simulink model "M_MSGPACKER"  (R2022a)
settings: Solver=ode4  StartTime=0.0  StopTime=0.04  FixedStep=0.04  RelTol=1e-3
PreLoadFcn:
  | listing = dir;
  | if (contains([listing .name], 'M_MSGPACKER.slx'))
  |     addpath('./DYN', './FLCC', './FTG', './GPS', './INS', './MAP', './RALT');
  | elseif (contains([listing .name], 'FTG.slx'))
  |     addpath('../DYN', '../FLCC', '../FTG', '../GPS', '../INS', '../MAP', '../RALT');
  | else
  | 
  | end
  | 
  | load('BUS_STRUCTURE_RALT.mat');
  | load('BUS_STRUCTURE_INS.mat');
  | load('BUS_STRUCTURE_GPS.mat');
InitFcn:
  | listing = dir;
  | if (contains([listing .name], 'M_MSGPACKER'))
  |     addpath('./DYN', './FLCC', './FTG', './GPS', './INS', './MAP', './RALT');
  | elseif (contains([listing .name], 'FTG.slx'))
  |     addpath('../DYN', '../FLCC', '../FTG', '../GPS', '../INS', '../MAP', '../RALT');
  | else
  | 
  | end
  | 
  | load('BUS_STRUCTURE_RALT.mat');
  | load('BUS_STRUCTURE_INS.mat');
  | load('BUS_STRUCTURE_GPS.mat');
undefined symbols (not defined in the file or in its folder): ft, m, s
libraries: aerolibconvert2 x14, simulink_extras x5
settings Model: Creator=ASCL  LastModifiedBy=ASCL
settings DataIOCC: SaveOutput=off  DSMLogging=off  SaveTime=off
settings OptimizationCC: BlockReduction=off  DefaultParameterBehavior=Inlined  UseDivisionForNetSlopeComputation=on  GainParamInheritBuiltInType=on  UseFloatMulNetSlope=on  ExpressionFolding=off  PassReuseOutputArgsAs=Individual arguments  ZeroExternalMemoryAtStartup=off  ZeroInternalMemoryAtStartup=off  EfficientFloat2IntCast=on  LifeSpan=inf  OptimizeBlockOrder=speed  DifferentSizesBufferReuse=on  EfficientTunableParamExpr=on
settings DebuggingCC: SignalInfNanChecking=warning  ReadBeforeWriteMsg=EnableAllAsError  WriteAfterWriteMsg=EnableAllAsError  WriteAfterReadMsg=EnableAllAsError  IntegerOverflowMsg=error  ParameterTunabilityLossMsg=error  UniqueDataStoreMsg=error  AssertControl=DisableAll  NonBusSignalsTreatedAsBus=error  SFInvalidInputDataAccessInChartInitDiag=error  SFTransitionOutsideNaturalParentDiag=error  SFUnreachableExecutionPathDiag=error  SFUndirectedBroadcastEventsDiag=error  IntegerSaturationMsg=error
settings HardwareCC: ProdBitPerPointer=32  ProdBitPerSizeT=32  ProdBitPerPtrDiffT=32  ProdLargestAtomicInteger=Long  ProdLargestAtomicFloat=Double  ProdEndianess=BigEndian  ProdWordSize=32  ProdLongLongMode=on  ProdHWDeviceType=Freescale->MPC83xx
settings ModelReferenceCC: ModelReferenceNumInstancesAllowed=Single
settings SFSimCC: CompileTimeRecursionLimit=0  EnableRuntimeRecursion=off  MATLABDynamicMemAlloc=off
settings RTWCC: SystemTargetFile=ert.tlc  TemplateMakefile=ert_default_tmf  GenerateReport=on  RTWUseSimCustomCode=on  BuildConfiguration=Faster Runs  IncludeHyperlinkInReport=on  LaunchReport=on  GenerateTraceInfo=on  GenerateTraceReport=on  GenerateTraceReportSl=on  GenerateTraceReportSf=on  GenerateTraceReportEml=on  GenerateCodeMetricsReport=on
settings CodeAppCC: ForceParamTrailComments=on  IgnoreCustomStorageClasses=off  OperatorAnnotations=on  SimulinkDataObjDesc=on  SFDataObjDesc=on  MATLABFcnDesc=on  InsertBlockDesc=on  StateflowObjectComments=on  MATLABSourceComments=on  EnableCustomComments=on  InlinedPrmAccess=Macros  ReqsInCode=on
settings ERTTargetCC: TargetLangStandard=C99 (ISO)  UtilityFuncGeneration=Shared location  GenerateSampleERTMain=on  IncludeMdlTerminateFcn=off  CombineSignalStateStructs=on  SuppressErrorStatus=on  SupportAbsoluteTime=off  SupportNonFinite=off  SupportComplex=off  ParenthesesLevel=Standards  CastingMode=Standards  GenerateSharedConstants=off  InlinedParameterPlacement=NonHierarchical  ERTCustomFileTemplate=example_file_process.tlc  RateTransitionBlockCode=Function  PreserveIfCondition=on  ConvertIfToSwitch=off  EnableSignedLeftShifts=off  EnableSignedRightShifts=off

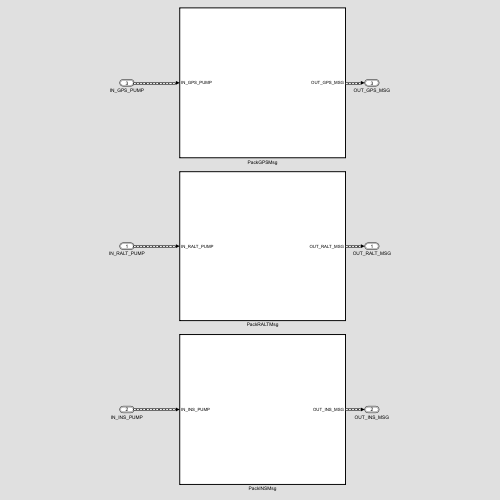
[thumbnail: Simulink's stored preview of the top-level diagram]
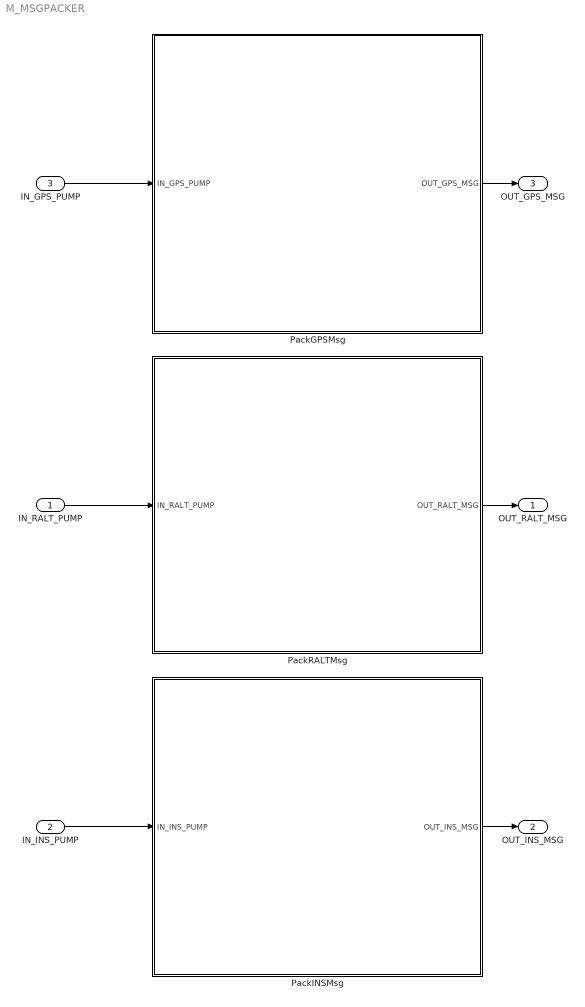
== system M_MSGPACKER ==
  IN_RALT_PUMP : Inport  OutDataTypeStr=Bus: BUS_SENSOR_RALT_DP  SampleTime=0.04  Interpolate=off  BusOutputAsStruct=on
  IN_INS_PUMP : Inport  Port=2  OutDataTypeStr=Bus: BUS_SENSOR_INS_DP  SampleTime=0.04  Interpolate=off  BusOutputAsStruct=on
  IN_GPS_PUMP : Inport  Port=3  OutDataTypeStr=Bus: BUS_SENSOR_GPS_DP  SampleTime=0.04  Interpolate=off  BusOutputAsStruct=on
  PackGPSMsg : Subsystem  TreatAsAtomicUnit=on
      settings: RTWSystemCode=Nonreusable function  RTWFcnNameOpts=Use subsystem name  FunctionInterfaceSpec=Allow arguments (Match graphical interface)
  PackINSMsg : Subsystem  TreatAsAtomicUnit=on
      settings: RTWSystemCode=Nonreusable function  RTWFcnNameOpts=Use subsystem name  FunctionInterfaceSpec=Allow arguments (Match graphical interface)
  PackRALTMsg : Subsystem  TreatAsAtomicUnit=on
      settings: RTWSystemCode=Nonreusable function  RTWFcnNameOpts=Use subsystem name  FunctionInterfaceSpec=Allow arguments (Match graphical interface)
  OUT_RALT_MSG : Outport  OutDataTypeStr=Bus: BUS_SENSOR_RALT  SampleTime=0.04  BusOutputAsStruct=on
  OUT_INS_MSG : Outport  Port=2  OutDataTypeStr=Bus: BUS_SENSOR_INS  SampleTime=0.04  BusOutputAsStruct=on
  OUT_GPS_MSG : Outport  Port=3  OutDataTypeStr=Bus: BUS_SENSOR_GPS  SampleTime=0.04  BusOutputAsStruct=on
  wires:
  IN_INS_PUMP/1 -> PackINSMsg/1(IN_INS_PUMP)
  PackGPSMsg/1(OUT_GPS_MSG) -> OUT_GPS_MSG/1
  IN_GPS_PUMP/1 -> PackGPSMsg/1(IN_GPS_PUMP)
  PackINSMsg/1(OUT_INS_MSG) -> OUT_INS_MSG/1
  PackRALTMsg/1(OUT_RALT_MSG) -> OUT_RALT_MSG/1
  IN_RALT_PUMP/1 -> PackRALTMsg/1(IN_RALT_PUMP)

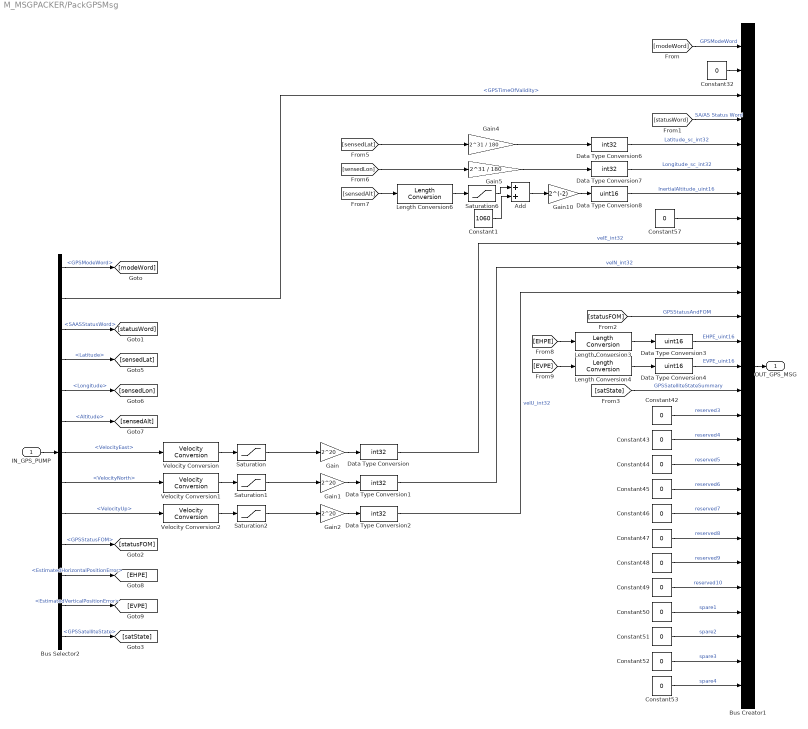
== system M_MSGPACKER/PackGPSMsg ==
  IN_GPS_PUMP : Inport  OutDataTypeStr=Bus: BUS_SENSOR_GPS_DP  SampleTime=0.04
  Add : Sum
  Bus Creator1 : BusCreator  Inputs=27  OutDataTypeStr=Bus: BUS_SENSOR_GPS  NonVirtualBus=on
      settings: InheritFromInputs=off
  Bus Selector2 : BusSelector  OutputSignals=GPSModeWord,GPSTimeOfValidity,SAASStatusWord,Latitude,Longitude,Altitude,VelocityEast,VelocityNorth,VelocityUp,GPSStatusFOM,EstimatedHorizontalPositionError,EstimatedVerticalPositionError,GPSSatelliteState
  Constant1 : Constant  Value=1060  SampleTime=0.04
  Constant{32,42..53,57} (14 alike) : Constant  Value=0  OutDataTypeStr=uint16  SampleTime=0.04
  Data Type Conversion{,1..2,6..7} (5 alike) : DataTypeConversion  OutDataTypeStr=int32  SaturateOnIntegerOverflow=off  RndMeth=Floor
  Data Type Conversion3 : DataTypeConversion  OutDataTypeStr=uint16  SaturateOnIntegerOverflow=off  RndMeth=Floor
  Data Type Conversion4 : DataTypeConversion  OutDataTypeStr=uint16  SaturateOnIntegerOverflow=off  RndMeth=Floor
  Data Type Conversion8 : DataTypeConversion  OutDataTypeStr=uint16  SaturateOnIntegerOverflow=off  RndMeth=Floor
  Gain : Gain  Gain=2^20
  Gain1 : Gain  Gain=2^20
  Gain10 : Gain  Gain=2^(-2)
  Gain2 : Gain  Gain=2^20
  Gain4 : Gain  Gain=2^31 / 180
  Gain5 : Gain  Gain=2^31 / 180
  Length Conversion3 : aerolibconvert2/Length Conversion  IU=m  OU=ft
  Length Conversion4 : aerolibconvert2/Length Conversion  IU=m  OU=ft
  Length Conversion6 : aerolibconvert2/Length Conversion  IU=m  OU=ft
  Saturation : Saturate  UpperLimit=2048  LowerLimit=-2048
  Saturation1 : Saturate  UpperLimit=2048  LowerLimit=-2048
  Saturation2 : Saturate  UpperLimit=2048  LowerLimit=-2048
  Saturation6 : Saturate  UpperLimit=80337  LowerLimit=-1060
  Velocity Conversion : aerolibconvert2/Velocity Conversion  IU=m/s  OU=ft/s
  Velocity Conversion1 : aerolibconvert2/Velocity Conversion  IU=m/s  OU=ft/s
  Velocity Conversion2 : aerolibconvert2/Velocity Conversion  IU=m/s  OU=ft/s
  OUT_GPS_MSG : Outport  SampleTime=0.04
  wires:
  Bus Creator1/1 -> OUT_GPS_MSG/1
  Data Type Conversion8/1 -> Bus Creator1/7  "InertialAltitude_uint16"
  Constant49/1 -> Bus Creator1/23  "reserved10"
  Gain4/1 -> Data Type Conversion6/1
  Constant44/1 -> Bus Creator1/18  "reserved5"
  [statusWord] -> Bus Creator1/4  "SA/AS Status Word"
  Gain5/1 -> Data Type Conversion7/1
  Constant1/1 -> Add/2
  Constant42/1 -> Bus Creator1/16  "reserved3"
  Constant46/1 -> Bus Creator1/20  "reserved7"
  Data Type Conversion4/1 -> Bus Creator1/14  "EVPE_uint16"
  Constant53/1 -> Bus Creator1/27  "spare4"
  Data Type Conversion3/1 -> Bus Creator1/13  "EHPE_uint16"
  Constant50/1 -> Bus Creator1/24  "spare1"
  [EVPE] -> Length Conversion4/1
  Velocity Conversion2/1 -> Saturation2/1
  Data Type Conversion6/1 -> Bus Creator1/5  "Latitude_sc_int32"
  Gain/1 -> Data Type Conversion/1
  [sensedLat] -> Gain4/1
  Constant52/1 -> Bus Creator1/26  "spare3"
  Constant47/1 -> Bus Creator1/21  "reserved8"
  Data Type Conversion7/1 -> Bus Creator1/6  "Longitude_sc_int32"
  Constant32/1 -> Bus Creator1/2
  Constant57/1 -> Bus Creator1/8
  Gain10/1 -> Data Type Conversion8/1
  Constant45/1 -> Bus Creator1/19  "reserved6"
  [satState] -> Bus Creator1/15  "GPSSatelliteStateSummary"
  Saturation6/1 -> Add/1
  Constant48/1 -> Bus Creator1/22  "reserved9"
  [statusFOM] -> Bus Creator1/12  "GPSStatusAndFOM"
  Gain1/1 -> Data Type Conversion1/1
  Velocity Conversion/1 -> Saturation/1
  Constant43/1 -> Bus Creator1/17  "reserved4"
  Length Conversion3/1 -> Data Type Conversion3/1
  Constant51/1 -> Bus Creator1/25  "spare2"
  Add/1 -> Gain10/1
  [sensedLon] -> Gain5/1
  Data Type Conversion/1 -> Bus Creator1/9  "velE_int32"
  Data Type Conversion2/1 -> Bus Creator1/11  "velU_int32"
  Data Type Conversion1/1 -> Bus Creator1/10  "velN_int32"
  Saturation1/1 -> Gain1/1
  Length Conversion4/1 -> Data Type Conversion4/1
  Gain2/1 -> Data Type Conversion2/1
  Velocity Conversion1/1 -> Saturation1/1
  Saturation2/1 -> Gain2/1
  [modeWord] -> Bus Creator1/1  "GPSModeWord"
  [sensedAlt] -> Length Conversion6/1
  Saturation/1 -> Gain/1
  [EHPE] -> Length Conversion3/1
  Length Conversion6/1 -> Saturation6/1
  IN_GPS_PUMP/1 -> Bus Selector2/1
  Bus Selector2/13 -> [satState]  "<GPSSatelliteState>"
  Bus Selector2/12 -> [EVPE]  "<EstimatedVerticalPositionError>"
  Bus Selector2/11 -> [EHPE]  "<EstimatedHorizontalPositionError>"
  Bus Selector2/10 -> [statusFOM]  "<GPSStatusFOM>"
  Bus Selector2/9 -> Velocity Conversion2/1  "<VelocityUp>"
  Bus Selector2/8 -> Velocity Conversion1/1  "<VelocityNorth>"
  Bus Selector2/7 -> Velocity Conversion/1  "<VelocityEast>"
  Bus Selector2/6 -> [sensedAlt]  "<Altitude>"
  Bus Selector2/5 -> [sensedLon]  "<Longitude>"
  Bus Selector2/4 -> [sensedLat]  "<Latitude>"
  Bus Selector2/3 -> [statusWord]  "<SAASStatusWord>"
  Bus Selector2/1 -> [modeWord]  "<GPSModeWord>"
  Bus Selector2/2 -> Bus Creator1/3  "<GPSTimeOfValidity>"

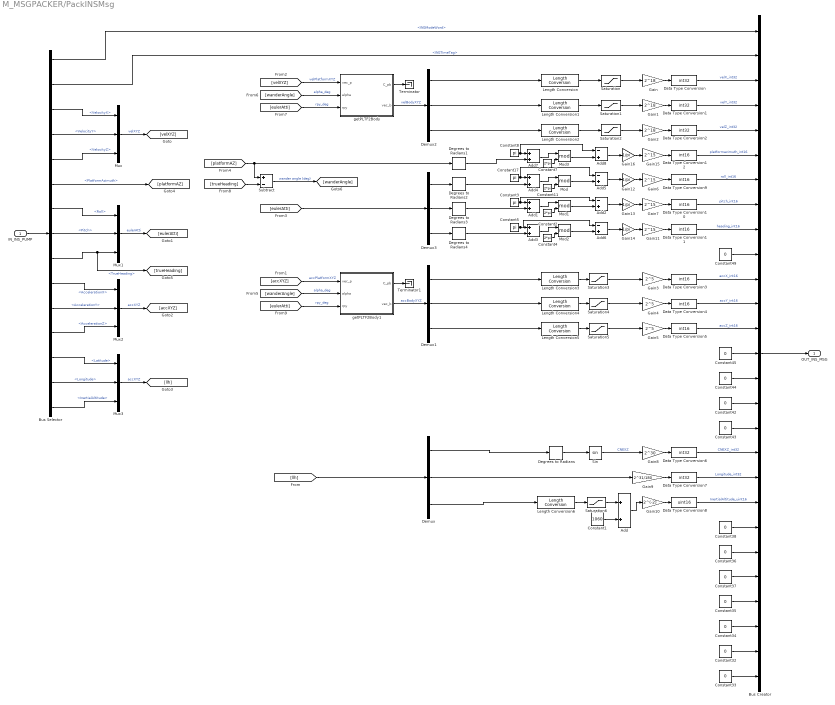
== system M_MSGPACKER/PackINSMsg ==
  IN_INS_PUMP : Inport  OutDataTypeStr=Bus: BUS_SENSOR_INS_DP  SampleTime=0.04
  Add{,1,3..4,7} (5 alike) : Sum
  Add{2,5..6,8} (4 alike) : Sum  Inputs=-+
  Bus Creator : BusCreator  Inputs=27  OutDataTypeStr=Bus: BUS_SENSOR_INS  NonVirtualBus=on
      settings: InheritFromInputs=off
  Bus Selector : BusSelector  OutputSignals=INSModeWord,INSTimeTag,VelocityX,VelocityY,VelocityZ,PlatformAzimuth,Roll,Pitch,TrueHeading,AccelerationX,AccelerationY,AccelerationZ,Latitude,Longitude,InertialAltitude
  Constant1 : Constant  Value=1060  SampleTime=0.04
  Constant{2,4,7,11} (4 alike) : Constant  Value=2*pi  SampleTime=0.04
  Constant{3,5,8,17} (4 alike) : Constant  Value=pi  SampleTime=0.04
  Constant{32..34,36..38,42..45,49} (11 alike) : Constant  Value=0  OutDataTypeStr=int16  SampleTime=0.04
  Constant35 : Constant  Value=0  OutDataTypeStr=uint16  SampleTime=0.04
  Data Type Conversion{,1..2,6..7} (5 alike) : DataTypeConversion  OutDataTypeStr=int32  SaturateOnIntegerOverflow=off  RndMeth=Floor
  Data Type Conversion{3..5,9..12} (7 alike) : DataTypeConversion  OutDataTypeStr=int16  SaturateOnIntegerOverflow=off  RndMeth=Floor
  Data Type Conversion8 : DataTypeConversion  OutDataTypeStr=uint16  SaturateOnIntegerOverflow=off  RndMeth=Floor
  Degrees to Radians{,1..4} (5 alike) : simulink_extras/Transformations/Degrees to Radians
  Demux{,1..3} (4 alike) : Demux  Outputs=3
  Gain : Gain  Gain=2^18
  Gain1 : Gain  Gain=2^18
  Gain10 : Gain  Gain=2^(-2)
  Gain{6..7,11,15} (4 alike) : Gain  Gain=2^15
  Gain{12..14,16} (4 alike) : Gain  Gain=1/pi
  Gain2 : Gain  Gain=2^18
  Gain3 : Gain  Gain=2^5
  Gain4 : Gain  Gain=2^5
  Gain5 : Gain  Gain=2^5
  Gain8 : Gain  Gain=2^30
  Gain9 : Gain  Gain=2^31/180
  Length Conversion{,1..6} (7 alike) : aerolibconvert2/Length Conversion  IU=m  OU=ft
  Mod{,1..3} (4 alike) : Math  Operator=mod
  Mux{,1..3} (4 alike) : Mux  Inputs=3
  Saturation : Saturate  UpperLimit=3000  LowerLimit=-3000
  Saturation1 : Saturate  UpperLimit=3000  LowerLimit=-3000
  Saturation2 : Saturate  UpperLimit=3000  LowerLimit=-3000
  Saturation3 : Saturate  UpperLimit=512  LowerLimit=-512
  Saturation4 : Saturate  UpperLimit=512  LowerLimit=-512
  Saturation5 : Saturate  UpperLimit=512  LowerLimit=-512
  Saturation6 : Saturate  UpperLimit=80337  LowerLimit=-1060
  Sin : Trigonometry
  Subtract : Sum  Inputs=+-
  Terminator : Terminator
  Terminator1 : Terminator
  getPLTF2Body : MATLAB Function  TreatAsAtomicUnit=on  SystemSampleTime=0.04
  getPLTF2Body1 : MATLAB Function  TreatAsAtomicUnit=on  SystemSampleTime=0.04
  OUT_INS_MSG : Outport  SampleTime=0.04
  wires:
  Bus Creator/1 -> OUT_INS_MSG/1
  Constant42/1 -> Bus Creator/16
  Data Type Conversion3/1 -> Bus Creator/11  "accX_int16"
  Constant44/1 -> Bus Creator/15
  Data Type Conversion6/1 -> Bus Creator/18  "CNEXZ_int32"
  Constant37/1 -> Bus Creator/23
  Data Type Conversion9/1 -> Bus Creator/7  "roll_int16"
  Constant36/1 -> Bus Creator/22
  Gain2/1 -> Data Type Conversion2/1
  Constant38/1 -> Bus Creator/21
  Length Conversion4/1 -> Saturation4/1
  Length Conversion1/1 -> Saturation1/1
  Length Conversion3/1 -> Saturation3/1
  Constant33/1 -> Bus Creator/27
  Constant35/1 -> Bus Creator/24
  Constant34/1 -> Bus Creator/25
  Bus Selector/1 -> Bus Creator/1  "<INSModeWord>"
  Data Type Conversion8/1 -> Bus Creator/20  "InertialAltitude_uint16"
  Data Type Conversion2/1 -> Bus Creator/5  "velZ_int32"
  Constant32/1 -> Bus Creator/26
  Add7/1 -> Mod3/1
  Gain1/1 -> Data Type Conversion1/1
  Demux/1 -> Degrees to Radians/1
  Demux2/3 -> Length Conversion2/1
  Demux/3 -> Length Conversion6/1
  Demux1/1 -> Length Conversion3/1
  Length Conversion5/1 -> Saturation5/1
  Demux/2 -> Gain9/1
  Data Type Conversion1/1 -> Bus Creator/4  "velY_int32"
  Degrees to Radians/1 -> Sin/1
  Demux1/2 -> Length Conversion4/1
  Gain13/1 -> Gain7/1
  Constant45/1 -> Bus Creator/14
  Data Type Conversion5/1 -> Bus Creator/13  "accZ_int16"
  Data Type Conversion11/1 -> Bus Creator/9  "heading_int16"
  [eulerAtti] -> Demux3/1
  Data Type Conversion4/1 -> Bus Creator/12  "accY_int16"
  [platformAZ] -> Subtract/1, Degrees to Radians1/1
  Demux3/1 -> Degrees to Radians2/1
  Demux3/3 -> Degrees to Radians4/1
  Demux3/2 -> Degrees to Radians3/1
  Gain15/1 -> Data Type Conversion12/1
  Constant8/1 -> Add8/1, Add7/1
  Length Conversion2/1 -> Saturation2/1
  Constant11/1 -> Mod/2
  Saturation4/1 -> Gain4/1
  Add4/1 -> Mod/1
  Demux2/1 -> Length Conversion/1
  Saturation1/1 -> Gain1/1
  [llh] -> Demux/1
  Demux2/2 -> Length Conversion1/1
  Mod/1 -> Add5/2
  Demux1/3 -> Length Conversion5/1
  Add5/1 -> Gain12/1
  Gain14/1 -> Gain11/1
  Constant7/1 -> Mod3/2
  Mod3/1 -> Add8/2
  Gain11/1 -> Data Type Conversion11/1
  Add3/1 -> Mod2/1
  Gain12/1 -> Gain6/1
  Add6/1 -> Gain14/1
  Data Type Conversion12/1 -> Bus Creator/6  "platformazimuth_int16"
  [velXYZ] -> getPLTF2Body/1(vec_p)  "velPlatformXYZ"
  Mod2/1 -> Add6/2
  getPLTF2Body1/2(vec_b) -> Demux1/1  "accBodyXYZ"
  [accXYZ] -> getPLTF2Body1/1(vec_p)  "accPlatformXYZ"
  Gain9/1 -> Data Type Conversion7/1
  Saturation3/1 -> Gain3/1
  Gain7/1 -> Data Type Conversion10/1
  Gain3/1 -> Data Type Conversion3/1
  Data Type Conversion10/1 -> Bus Creator/8  "pitch_int16"
  Add1/1 -> Mod1/1
  Constant4/1 -> Mod2/2
  Data Type Conversion7/1 -> Bus Creator/19  "Longitude_int32"
  Saturation2/1 -> Gain2/1
  Constant3/1 -> Add1/1, Add2/1
  Constant1/1 -> Add/2
  Constant2/1 -> Mod1/2
  Sin/1 -> Gain8/1  "CNEXZ"
  Add2/1 -> Gain13/1
  Gain16/1 -> Gain15/1
  Constant5/1 -> Add6/1, Add3/1
  Mod1/1 -> Add2/2
  Gain6/1 -> Data Type Conversion9/1
  Saturation/1 -> Gain/1
  Add8/1 -> Gain16/1
  Constant17/1 -> Add5/1, Add4/1
  Constant49/1 -> Bus Creator/10
  Gain5/1 -> Data Type Conversion5/1
  Add/1 -> Gain10/1
  Constant43/1 -> Bus Creator/17
  Length Conversion/1 -> Saturation/1
  Gain/1 -> Data Type Conversion/1
  Data Type Conversion/1 -> Bus Creator/3  "velX_int32"
  Saturation5/1 -> Gain5/1
  Saturation6/1 -> Add/1
  Gain10/1 -> Data Type Conversion8/1
  Gain8/1 -> Data Type Conversion6/1
  Gain4/1 -> Data Type Conversion4/1
  Length Conversion6/1 -> Saturation6/1
  IN_INS_PUMP/1 -> Bus Selector/1
  Bus Selector/2 -> Bus Creator/2  "<INSTimeTag>"
  Bus Selector/3 -> Mux/1  "<VelocityX>"
  Bus Selector/4 -> Mux/2  "<VelocityY>"
  Bus Selector/5 -> Mux/3  "<VelocityZ>"
  Bus Selector/6 -> [platformAZ]  "<PlatformAzimuth>"
  Bus Selector/7 -> Mux1/1  "<Roll>"
  Bus Selector/8 -> Mux1/2  "<Pitch>"
  Bus Selector/9 -> [trueHeading], Mux1/3  "<TrueHeading>"
  Bus Selector/10 -> Mux2/1  "<AccelerationX>"
  Bus Selector/11 -> Mux2/2  "<AccelerationY>"
  Bus Selector/12 -> Mux2/3  "<AccelerationZ>"
  Bus Selector/13 -> Mux3/1  "<Latitude>"
  Bus Selector/14 -> Mux3/2  "<Longitude>"
  Bus Selector/15 -> Mux3/3  "<InertialAltitude>"
  Mux/1 -> [velXYZ]  "velXYZ"
  Mux1/1 -> [eulerAtti]  "eulerAtti"
  Mux2/1 -> [accXYZ]  "accXYZ"
  Mux3/1 -> [llh]  "accXYZ"
  Degrees to Radians1/1 -> Add7/2
  Degrees to Radians2/1 -> Add4/2
  Degrees to Radians3/1 -> Add1/2
  Degrees to Radians4/1 -> Add3/2
  [eulerAtti] -> getPLTF2Body/3(rpy)  "rpy_deg"
  [trueHeading] -> Subtract/2
  Subtract/1 -> [wanderAngle]  "wander angle (deg)"
  [wanderAngle] -> getPLTF2Body/2(alpha)  "alpha_deg"
  [wanderAngle] -> getPLTF2Body1/2(alpha)  "alpha_deg"
  [eulerAtti] -> getPLTF2Body1/3(rpy)  "rpy_deg"
  getPLTF2Body1/1(C_pb) -> Terminator1/1
  getPLTF2Body/1(C_pb) -> Terminator/1
  getPLTF2Body/2(vec_b) -> Demux2/1  "velBodyXYZ"

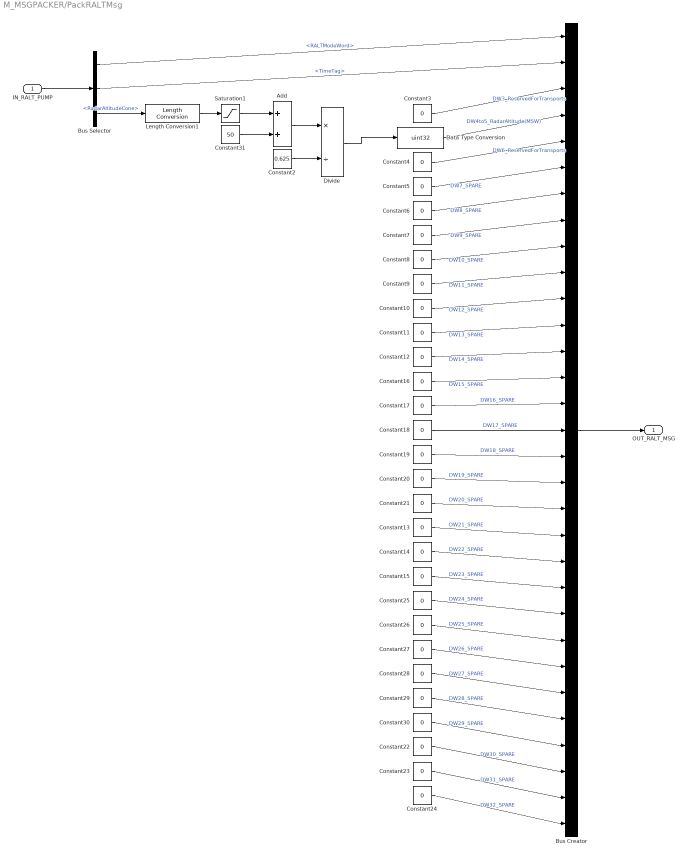
== system M_MSGPACKER/PackRALTMsg ==
  IN_RALT_PUMP : Inport  OutDataTypeStr=Bus: BUS_SENSOR_RALT_DP  SampleTime=0.04
  Add : Sum
  Bus Creator : BusCreator  Inputs=31  OutDataTypeStr=Bus: BUS_SENSOR_RALT  NonVirtualBus=on
      settings: InheritFromInputs=off
  Bus Selector : BusSelector  OutputSignals=RALTModeWord,TimeTag,RadarAltitudeCone
  Constant{3..13,15..30} (27 alike) : Constant  Value=0  OutDataTypeStr=uint16  SampleTime=0.04
  Constant14 : Constant  Value=0  OutDataTypeStr=uint16
  Constant2 : Constant  Value=0.625  SampleTime=0.04
  Constant31 : Constant  Value=50  SampleTime=0.04
  Data Type Conversion : DataTypeConversion  OutDataTypeStr=uint32  RndMeth=Round  SaturateOnIntegerOverflow=off
  Divide : Product  Inputs=*/
  Length Conversion1 : aerolibconvert2/Length Conversion  IU=m  OU=ft
  Saturation1 : Saturate  UpperLimit=50000  LowerLimit=-50
  OUT_RALT_MSG : Outport  SampleTime=0.04
  wires:
  Add/1 -> Divide/1
  Constant31/1 -> Add/2
  Divide/1 -> Data Type Conversion/1
  Constant24/1 -> Bus Creator/31  "DW32_SPARE"
  Length Conversion1/1 -> Saturation1/1
  Constant17/1 -> Bus Creator/15  "DW16_SPARE"
  Constant11/1 -> Bus Creator/12  "DW13_SPARE"
  Constant19/1 -> Bus Creator/17  "DW18_SPARE"
  Saturation1/1 -> Add/1
  Constant29/1 -> Bus Creator/27  "DW28_SPARE"
  Constant16/1 -> Bus Creator/14  "DW15_SPARE"
  Constant23/1 -> Bus Creator/30  "DW31_SPARE"
  Constant21/1 -> Bus Creator/19  "DW20_SPARE"
  Constant9/1 -> Bus Creator/10  "DW11_SPARE"
  Constant27/1 -> Bus Creator/25  "DW26_SPARE"
  Constant10/1 -> Bus Creator/11  "DW12_SPARE"
  Constant20/1 -> Bus Creator/18  "DW19_SPARE"
  Constant28/1 -> Bus Creator/26  "DW27_SPARE"
  Constant14/1 -> Bus Creator/21  "DW22_SPARE"
  Constant13/1 -> Bus Creator/20  "DW21_SPARE"
  Constant26/1 -> Bus Creator/24  "DW25_SPARE"
  Constant15/1 -> Bus Creator/22  "DW23_SPARE"
  Constant25/1 -> Bus Creator/23  "DW24_SPARE"
  Constant18/1 -> Bus Creator/16  "DW17_SPARE"
  Constant8/1 -> Bus Creator/9  "DW10_SPARE"
  Constant7/1 -> Bus Creator/8  "DW9_SPARE"
  Constant12/1 -> Bus Creator/13  "DW14_SPARE"
  Constant6/1 -> Bus Creator/7  "DW8_SPARE"
  Bus Creator/1 -> OUT_RALT_MSG/1
  Bus Selector/2 -> Bus Creator/2  "<TimeTag>"
  Constant30/1 -> Bus Creator/28  "DW29_SPARE"
  Constant4/1 -> Bus Creator/5  "DW6_ReservedForTransports"
  Bus Selector/3 -> Length Conversion1/1  "<RadarAltitudeCone>"
  Constant3/1 -> Bus Creator/3  "DW3_ReservedForTransports"
  Constant22/1 -> Bus Creator/29  "DW30_SPARE"
  Constant5/1 -> Bus Creator/6  "DW7_SPARE"
  Constant2/1 -> Divide/2
  Data Type Conversion/1 -> Bus Creator/4  "DW4to5_RadarAltitude(MSW)"
  Bus Selector/1 -> Bus Creator/1  "<RALTModeWord>"
  IN_RALT_PUMP/1 -> Bus Selector/1

== matlab function M_MSGPACKER/PackINSMsg/getPLTF2Body1 ==
  data: vec_p input; C_pb output; alpha input; rpy input; vec_b output
function [C_pb, vec_b] = getPLTF2Body(vec_p, alpha, rpy)
%getPLTF2Body Convert a vector in INS Platform axis to body frame
%
% Inputs
%   vec_p   : a vector in INS platform axis (3x1)
%   alpha   : wander angle "platform azimuth - true heading" (deg)
%   rpy     : roll, pitch, yaw(true heading) angles (deg)
%
% Outputs
%   C_pb    : computed tranformation matrix from INS Platform axis to body 
% axis
%   vec_b   : converted vec_p in in body frame

% Initialize
C_pb = zeros(3,3);
vec_b = zeros(3,1);

% Arrange
cRol = cosd(rpy(1));
sRol = sind(rpy(1));
cPit = cosd(rpy(2));
sPit = sind(rpy(2));
cYaw = cosd(rpy(3));
sYaw = sind(rpy(3));

% Transformation matrix form INS Platform axis to local NED navigation
% frame
C_pn = [ cosd(alpha), -sind(alpha),  0; ...
        -sind(alpha), -cosd(alpha),  0; ...
                   0,            0, -1];

% Transformation matrix from local NED to body
C_nb = [               cPit*cYaw,                cPit*sYaw,     -sPit;...
        sRol*sPit*cYaw-cRol*sYaw, sRol*sPit*sYaw+cRol*cYaw, sRol*cPit;...
        cRol*sPit*cYaw+sRol*sYaw, cRol*sPit*sYaw-sRol*cYaw, cRol*cPit];

C_pb = C_nb * C_pn;

% Convert a given vector to body
vec_b = C_pb * vec_p;

end

== matlab function M_MSGPACKER/PackINSMsg/getPLTF2Body ==
  data: vec_p input; C_pb output; alpha input; rpy input; vec_b output
function [C_pb, vec_b] = getPLTF2Body(vec_p, alpha, rpy)
%getPLTF2Body Convert a vector in INS Platform axis to body frame
%
% Inputs
%   vec_p   : a vector in INS platform axis (3x1)
%   alpha   : wander angle "platform azimuth - true heading" (deg)
%   rpy     : roll, pitch, yaw(true heading) angles (deg)
%
% Outputs
%   C_pb    : computed tranformation matrix from INS Platform axis to body 
% axis
%   vec_b   : converted vec_p in in body frame

% Initialize
C_pb = zeros(3,3);
vec_b = zeros(3,1);

% Arrange
cRol = cosd(rpy(1));
sRol = sind(rpy(1));
cPit = cosd(rpy(2));
sPit = sind(rpy(2));
cYaw = cosd(rpy(3));
sYaw = sind(rpy(3));

% Transformation matrix form INS Platform axis to local NED navigation
% frame
C_pn = [ cosd(alpha), -sind(alpha),  0; ...
        -sind(alpha), -cosd(alpha),  0; ...
                   0,            0, -1];

% Transformation matrix from local NED to body
C_nb = [               cPit*cYaw,                cPit*sYaw,     -sPit;...
        sRol*sPit*cYaw-cRol*sYaw, sRol*sPit*sYaw+cRol*cYaw, sRol*cPit;...
        cRol*sPit*cYaw+sRol*sYaw, cRol*sPit*sYaw-sRol*cYaw, cRol*cPit];

C_pb = C_nb * C_pn;

% Convert a given vector to body
vec_b = C_pb * vec_p;

end
